simulink model "PID_simulation"  (R2016b)
settings: Solver=VariableStepAuto  StartTime=0.0  StopTime=2  RelTol=1e-3
values from neighbouring files (symbols this model uses):
  a0 = (mb * lb + mw * l) * g / (Ib + mw * l^2)    (= 36.2179403821)    [model_parameters.m]
  a1 = -1 / (Ib + mw * l^2)    (= -166.716681671)    [model_parameters.m]
  a2 = -Cb / (Ib + mw * l^2)    (= -0.170051015305)    [model_parameters.m]
  a3 = Cw/(Ib + mw * l^2)    (= 0.00833583408356)    [model_parameters.m]
  b0 = -a0    (= -36.2179403821)    [model_parameters.m]
  b1 = (Ib + Iw + mw * l^2) / (Iw * (Ib + mw * l^2))    (= 537.087052042)    [model_parameters.m]
  b2 = -a2    (= 0.170051015305)    [model_parameters.m]
  b3 = -Cw * b1    (= -0.0268543526021)    [model_parameters.m]
  Km = 25.1e-3    (= 0.0251)    [model_parameters.m]
  maxDCCurrent = 10    [model_parameters.m]
  sampleTime = 0.01    [model_parameters.m]
undefined symbols (not defined in the file or in its folder): pidnn_link
libraries: simulink x1
settings Model: Creator=viraj  LastModifiedBy=viraj

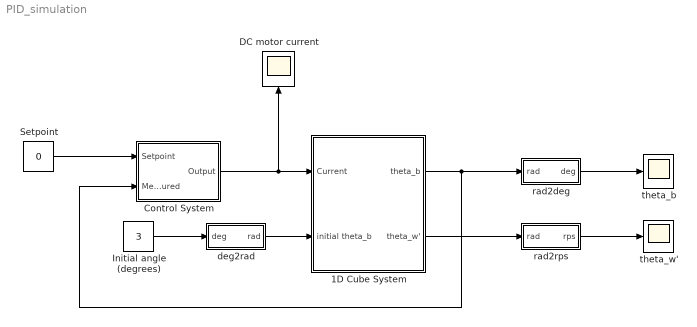
== system PID_simulation ==
  1D Cube System : Subsystem
  Control System : Subsystem
  DC motor current : Scope
  Initial angle (degrees) : Constant  Value=3
  Setpoint : Constant  Value=0
  deg2rad : Subsystem
  rad2deg : Subsystem
  rad2rps : Subsystem
  theta_b : Scope
  theta_w' : Scope
  wires:
  1D Cube System/1(theta_b) -> rad2deg/1(rad), Control System/2(Measured)
  deg2rad/1("rad ") -> 1D Cube System/2("initial theta_b ")
  rad2deg/1("deg ") -> theta_b/1
  Initial angle (degrees)/1 -> deg2rad/1(deg)
  1D Cube System/2(theta_w') -> rad2rps/1(rad)
  rad2rps/1(rps) -> theta_w'/1
  Control System/1(Output) -> 1D Cube System/1("Current "), DC motor current/1
  Setpoint/1 -> Control System/1(Setpoint)

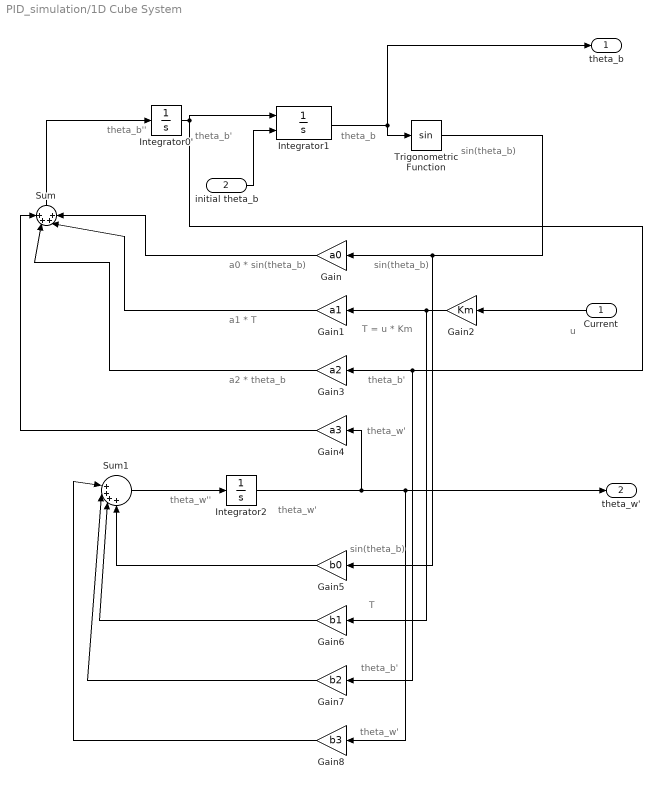
== system PID_simulation/1D Cube System ==
  note: theta_w'
  note: theta_b'
  note: T
  note: a2 * theta_b
  note: theta_b'
  note: sin(theta_b)
  note: theta_w'
  note: theta_w''
  note: T = u * Km
  note: u
  note: a1 * T
  note: a0 * sin(theta_b)
  note: sin(theta_b)
  note: theta_b''
  note: theta_b'
  note: theta_b
  note: sin(theta_b)
  note: theta_w'
  "Current " : Inport
  "initial theta_b " : Inport  Port=2
  Gain : Gain  Gain=a0
  Gain1 : Gain  Gain=a1
  Gain2 : Gain  Gain=Km
  Gain3 : Gain  Gain=a2
  Gain4 : Gain  Gain=a3
  Gain5 : Gain  Gain=b0
  Gain6 : Gain  Gain=b1
  Gain7 : Gain  Gain=b2
  Gain8 : Gain  Gain=b3
  Integrator0' : Integrator
  Integrator1 : Integrator  InitialConditionSource=external  InitialCondition=-0.1  LimitOutput=on  UpperSaturationLimit=pi  LowerSaturationLimit=-pi
  Integrator2 : Integrator
  Sum : Sum  Inputs=++++
  Sum1 : Sum  Inputs=||++++
  Trigonometric Function : Trigonometry
  theta_b : Outport
  theta_w' : Outport  Port=2
  wires:
  Gain1/1 -> Sum/3
  Trigonometric Function/1 -> Gain5/1, Gain/1
  Sum/1 -> Integrator0'/1
  Gain/1 -> Sum/4
  Integrator0'/1 -> Integrator1/1, Gain7/1, Gain3/1
  Integrator1/1 -> Trigonometric Function/1, theta_b/1
  Gain2/1 -> Gain1/1, Gain6/1
  "Current "/1 -> Gain2/1
  "initial theta_b "/1 -> Integrator1/2
  Gain3/1 -> Sum/2
  Integrator2/1 -> Gain8/1, theta_w'/1, Gain4/1
  Gain4/1 -> Sum/1
  Sum1/1 -> Integrator2/1
  Gain5/1 -> Sum1/4
  Gain6/1 -> Sum1/3
  Gain7/1 -> Sum1/2
  Gain8/1 -> Sum1/1

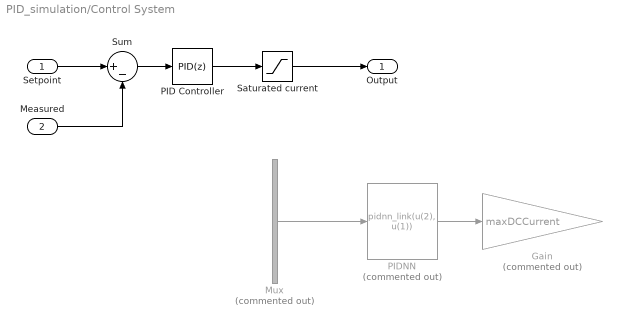
== system PID_simulation/Control System ==
  Setpoint : Inport
  Measured : Inport  Port=2
  Gain : Gain  Commented=on  Gain=maxDCCurrent
  Mux : Mux  Commented=on  Inputs=2
  PID Controller : simulink/Continuous/PID Controller  Controller=PID  TimeDomain=Discrete-time  SampleTime=sampleTime  IntegratorMethod=Forward Euler  FilterMethod=Forward Euler  Form=Parallel  UseFilter=off  ControllerParametersSource=internal  P=-79.9473716230485  I=-230  D=-8  N=179.879112686189  InitialConditionSource=internal  InitialConditionForIntegrator=0  InitialConditionForFilter=0  ExternalReset=none  LimitOutput=off  UpperSaturationLimit=inf  LowerSaturationLimit=-inf  LinearizeAsGain=on  AntiWindupMode=none  Kb=1  TrackingMode=off  Kt=1  PParamMin=[]  PParamMax=[]  IParamMin=[]  IParamMax=[]  DParamMin=[]  DParamMax=[]  NParamMin=[]  NParamMax=[]  KbParamMin=[]  KbParamMax=[]  KtParamMin=[]  KtParamMax=[]  POutMin=[]  POutMax=[]  IOutMin=[]  IOutMax=[]  DOutMin=[]  DOutMax=[]  NOutMin=[]  NOutMax=[]  KbOutMin=[]  KbOutMax=[]  KtOutMin=[]  KtOutMax=[]  IntegratorOutMin=[]  IntegratorOutMax=[]  FilterOutMin=[]  FilterOutMax=[]  SumOutMin=[]  SumOutMax=[]  SumI1OutMin=[]  SumI1OutMax=[]  SumI2OutMin=[]  SumI2OutMax=[]  SumI3OutMin=[]  SumI3OutMax=[]  SumDOutMin=[]  SumDOutMax=[]  SaturationOutMin=[]  SaturationOutMax=[]  IntegratorContinuousStateAttributes=''  IntegratorStateMustResolveToSignalObject=off  IntegratorRTWStateStorageClass=Auto  FilterContinuousStateAttributes=''  FilterStateMustResolveToSignalObject=off  FilterRTWStateStorageClass=Auto  DifferentiatorICPrevScaledInput=0  DifferentiatorOutMin=[]  DifferentiatorOutMax=[]
  PIDNN : MATLABFcn  Commented=on  MATLABFcn=pidnn_link(u(2), u(1))
  Saturated current : Saturate  UpperLimit=maxDCCurrent  LowerLimit=-maxDCCurrent
  Sum : Sum  Inputs=|+-
  Output : Outport
  wires:
  Sum/1 -> PID Controller/1
  PID Controller/1 -> Saturated current/1
  PIDNN/1 -> Gain/1
  Mux/1 -> PIDNN/1
  Measured/1 -> Sum/2
  Setpoint/1 -> Sum/1
  Saturated current/1 -> Output/1

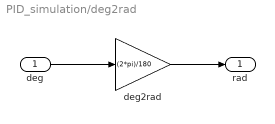
== system PID_simulation/deg2rad ==
  deg : Inport
  deg2rad : Gain  Gain=(2*pi)/180
  "rad " : Outport
  wires:
  deg/1 -> deg2rad/1
  deg2rad/1 -> "rad "/1

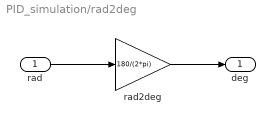
== system PID_simulation/rad2deg ==
  rad : Inport
  rad2deg : Gain  Gain=180/(2*pi)
  "deg " : Outport
  wires:
  rad/1 -> rad2deg/1
  rad2deg/1 -> "deg "/1

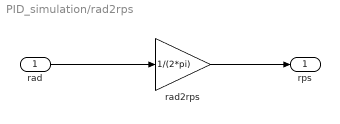
== system PID_simulation/rad2rps ==
  rad : Inport
  rad2rps : Gain  Gain=1/(2*pi)
  rps : Outport
  wires:
  rad/1 -> rad2rps/1
  rad2rps/1 -> rps/1
